simulink model "simulink_model_original"  (R2025a)
settings: Solver=VariableStepAuto  StartTime=0.0  StopTime=10.0  MaxStep=0.2  RelTol=1e-3  AbsTol=1e-3  EnableMultiTasking=on
libraries: fl_lib x8, nesl_utility x6, MyLib_lib x3, simulink x1
CloseFcn:
  | try,close(h1_MechanicalRotationalSystemWithStickSlipMotion),end
  | clear h1_MechanicalRotationalSystemWithStickSlipMotion
  | clear simlog_MechanicalRotationalSystemWithStickSlipMotion
Description:
  | Mechanical Rotational System with Stick-Slip Motion
settings Model: Creator=The MathWorks, Inc.  LastModifiedBy=tbe
settings SolverCC: AutoScaleAbsTol=off  AlgebraicLoopSolver=TrustRegion  MaxZcPerStep=1.0
settings DataIOCC: LimitDataPoints=on  SaveFormat=Array  ReturnWorkspaceOutputs=off
settings OptimizationCC: LifeSpan=inf
settings DebuggingCC: SolverPrmCheckMsg=warning  UnconnectedInputMsg=warning  UnconnectedOutputMsg=warning  UnconnectedLineMsg=warning  AllowSymbolicDim=off  PregeneratedLibrarySubsystemCodeDiagnostic=none  SFUnexpectedBacktrackingDiag=warning  SFNoUnconditionalDefaultTransitionDiag=warning  SFExecutionAtInitializationDiag=none  ArithmeticOperatorsInVariantConditions=warning
settings HardwareCC: ProdBitPerPointer=32.0  ProdBitPerSizeT=32.0  ProdBitPerPtrDiffT=32.0  ProdLargestAtomicFloat=None  ProdIntDivRoundTo=Undefined  ProdEndianess=Unspecified  ProdWordSize=32.0  ProdHWDeviceType=32-bit Generic
settings ModelReferenceCC: EnableRefExpFcnMdlSchedulingChecks=on  PropagateSignalLabelsOutOfModel=off
settings SFSimCC: SimUseLocalCustomCode=off  CustomCodeUndefinedFunction=UseInterfaceOnly
settings RTWCC: RTWUseLocalCustomCode=off  GPUComputeCapability=3.5  DLArmComputeVersion=19.05
settings CodeAppCC: StateflowObjectComments=on
settings GRTTargetCC: TargetLangStandard=C89/C90 (ANSI)
settings ConfigComp: CovMetricSettings=dw  CovSaveCumulativeToWorkspaceVar=on  CovSaveSingleToWorkspaceVar=on  CovExternalEMLEnable=off  CovSFcnEnable=off
settings SimscapeCC: SimscapeLogType=all  SimscapeLogSimulationStatistics=on  SimscapeLogName=simlog_MechanicalRotationalSystemWithStickSlipMotion  SimscapeLogDataHistory=10000.0

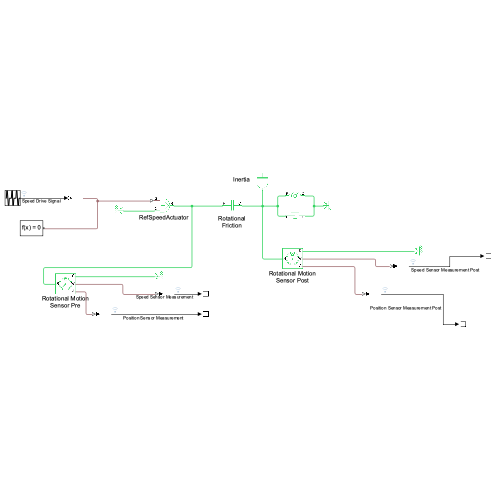
[thumbnail: Simulink's stored preview of the top-level diagram]
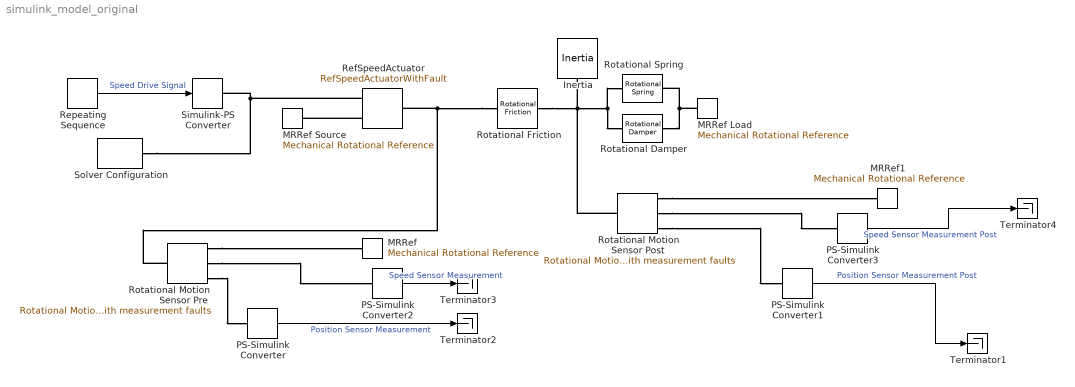
== system simulink_model_original ==
  Inertia : fl_lib/Mechanical/Rotational Elements/Inertia  Tag=Factory Generic  inertia=0.0001 kg*m^2  num_ports=foundation.enum.numPorts2.one  w_specify=off  w_priority=High  w=0 rad/s  w_nominal_specify=off  w_nominal_value=1  w_nominal_unit=rad/s  t_specify=off  t_priority=High  t=0 N*m  t_nominal_specify=off  t_nominal_value=1  t_nominal_unit=N*m
  MRRef : fl_lib/Mechanical/Rotational Elements/Mechanical Rotational Reference  Tag=Factory Generic
  MRRef Load : fl_lib/Mechanical/Rotational Elements/Mechanical Rotational Reference  Tag=Factory Generic
  MRRef Source : fl_lib/Mechanical/Rotational Elements/Mechanical Rotational Reference  Tag=Factory Generic
  MRRef1 : fl_lib/Mechanical/Rotational Elements/Mechanical Rotational Reference  Tag=Factory Generic
  PS-Simulink Converter{,1..3} (4 alike) : nesl_utility/PS-Simulink Converter  PhysicalDomain=network_engine_domain  SubClassName=ps_output  LeftPortType=input  RightPortType=output  PseudoPeriodic=off  Frequencies=[]  VectorFormat=1-D array  Unit=1  AffineConversion=off
  RefSpeedActuator : MyLib_lib/RefSpeedActuatorWithFault  fault_speed_bias=0 rad/s  fault_drift_rate=0 rad/s^2
      settings: InternalSimscapePortConfiguration="{\"Bottom\":[],\"Left\":[{\"id\":\"R\",\"label\":\"R\",\"type\":\"foundation.mechanical.rotational.rotational\"}],\"Right\":[{\"id\":\"S\",\"label\":\"S\",\"type\":\"input\"},{\"id\":\"C\",\"label\":\"C\",\"type\":\"foundation.mechanical.rotational.rotational\"}],\"Top\":[]}"
  Repeating Sequence : simulink/Sources/Repeating Sequence  rep_seq_t=[0 0.98 2 3 4.98 6 7 10]  rep_seq_y=[0 0 6 6 -6 -6 0 0]
  Rotational Friction : fl_lib/Mechanical/Rotational Elements/Rotational Friction  Tag=Factory Generic  brkwy_trq=25 m*N  brkwy_vel=0.06035 rad/s  Col_trq=20 m*N  visc_coef=0.001 m*s*N/rad  w_specify=off  w_priority=High  w=0 rad/s  w_nominal_specify=off  w_nominal_value=1  w_nominal_unit=rad/s  t_specify=off  t_priority=High  t=0 N*m  t_nominal_specify=off  t_nominal_value=1  t_nominal_unit=N*m
  Rotational Damper : fl_lib/Mechanical/Rotational Elements/Rotational Damper  Tag=Factory Generic  D=0.01 m*s*N/rad  w_specify=off  w_priority=High  w=0 rad/s  w_nominal_specify=off  w_nominal_value=1  w_nominal_unit=rad/s  t_specify=off  t_priority=High  t=0 N*m  t_nominal_specify=off  t_nominal_value=1  t_nominal_unit=N*m
  Rotational Motion Sensor Post : MyLib_lib/Rotational Motion Sensor with measurement faults  fault_speed_bias=0 rad/s  fault_speed_gain=0  fault_drift_rate=0 rad/s^2  fault_accel_bias=0 rad/s^2  reference=foundation.enum.MeasurementReference.difference  acceleration_port=false  velocity_port=true  position_port=true  wrap_angle=false  offset=0 rad
      settings: InternalSimscapePortConfiguration="{\"Bottom\":[],\"Left\":[{\"id\":\"R\",\"label\":\"R\",\"type\":\"foundation.mechanical.rotational.rotational\"}],\"Right\":[{\"id\":\"C\",\"label\":\"C\",\"type\":\"foundation.mechanical.rotational.rotational\"},{\"id\":\"W\",\"label\":\"W\",\"type\":\"output\"},{\"id\":\"A\",\"label\":\"A\",\"type\":\"output\"}],\"Top\":[]}"
  Rotational Motion Sensor Pre : MyLib_lib/Rotational Motion Sensor with measurement faults  fault_speed_bias=0 rad/s  fault_speed_gain=0  fault_drift_rate=0 rad/s^2  fault_accel_bias=0 rad/s^2  reference=foundation.enum.MeasurementReference.difference  acceleration_port=false  velocity_port=true  position_port=true  wrap_angle=false  offset=0 rad
      settings: InternalSimscapePortConfiguration="{\"Bottom\":[],\"Left\":[{\"id\":\"R\",\"label\":\"R\",\"type\":\"foundation.mechanical.rotational.rotational\"}],\"Right\":[{\"id\":\"C\",\"label\":\"C\",\"type\":\"foundation.mechanical.rotational.rotational\"},{\"id\":\"W\",\"label\":\"W\",\"type\":\"output\"},{\"id\":\"A\",\"label\":\"A\",\"type\":\"output\"}],\"Top\":[]}"
  Rotational Spring : fl_lib/Mechanical/Rotational Elements/Rotational Spring  Tag=Factory Generic  spr_rate=6.5 N*m/rad  w_specify=off  w_priority=High  w=0 rad/s  w_nominal_specify=off  w_nominal_value=1  w_nominal_unit=rad/s  t_specify=off  t_priority=High  t=0 N*m  t_nominal_specify=off  t_nominal_value=1  t_nominal_unit=N*m  phi_specify=off  phi_priority=High  phi=0 rad  phi_nominal_specify=off  phi_nominal_value=1  phi_nominal_unit=rad
  Simulink-PS Converter : nesl_utility/Simulink-PS Converter  PhysicalDomain=network_engine_domain  SubClassName=ps_input  LeftPortType=input  RightPortType=output  PseudoPeriodic=off  Frequencies=[]  NoiseDistribution=none  NoiseParameters=[]  Unit=1  AffineConversion=off  FilteringAndDerivatives=zero  SimscapeFilterOrder=1  InputFilterTimeConstant=.001  UdotUserProvided=[]
  Solver Configuration : nesl_utility/Solver Configuration  PhysicalDomain=network_engine_domain  SubClassName=solver  LeftPortType=input  RightPortType=generic  Tones=[]  Harmonics=[]  SimulateNoise=off  Profile=off  UseLocalSampling=off  EnableSwitchedLinearOptims=on  FrequencyDomain=off  UseCCode=off  RelTol=0.001  AbsTol=1e-06  MinStep=1e-09  ToWorkspace=off  RevertToSquareIcSolve=off  NumHomotopyIterations=100  PhasorMode=off  PhasorModeNumHarmonics=1  ConsistencySolver=NEWTON_XTOL_AFTER_FTOL  IndexReductionMethod=DerivativeReplacement  DoDC=off  ResidualTolerance=1e-9  ConsistencyTolSource=GLOBAL  ConsistencyAbsTol=0.001  ConsistencyRelTol=0.001  ConsistencyTolFactor=0.001  UseLocalSolver=off  LocalSolverChoice=NE_BACKWARD_EULER_ADVANCER  ResolveIndetEquations=on  FunctionEvalNumThread=1  LocalSolverSampleTime=.001  DoFixedCost=off  MaxNonlinIter=3  MaxModeIter=2  ComputeImpulses=off  ImpulseIterations=2  LinearAlgebra=auto  LinearAlgebraNumThread=0  EquationFormulation=NE_TIME_EF  DelaysMemoryBudget=1024  AutomaticFiltering=on  FilteringTimeConstant=0.001  PartitionStorageMethod=AS_NEEDED  PartitionMemoryBudget=1024  PartitionMethod=FAST  MultibodyUseLocalSolver=off  MultibodyLocalSolverChoice=ODE1  MultibodyLocalSolverSampleTime=0.001
  Terminator{1..4} (4 alike) : Terminator
  wires:
  PS-Simulink Converter/1 -> Terminator2/1  "Position Sensor Measurement"
  PS-Simulink Converter1/1 -> Terminator1/1  "Position Sensor Measurement Post"
  Repeating Sequence/1 -> Simulink-PS Converter/1  "Speed Drive Signal"
  PS-Simulink Converter2/1 -> Terminator3/1  "Speed Sensor Measurement"
  PS-Simulink Converter3/1 -> Terminator4/1  "Speed Sensor Measurement Post"
  connections:
  Rotational Spring/RConn1 -- MRRef Load/LConn1 -- Rotational Damper/RConn1
  Inertia/LConn1 -- Rotational Motion Sensor Post/LConn1 -- Rotational Friction/RConn1 -- Rotational Spring/LConn1 -- Rotational Damper/LConn1
  Rotational Friction/LConn1 -- Rotational Motion Sensor Pre/LConn1 -- RefSpeedActuator/LConn1
  RefSpeedActuator/RConn2 -- MRRef Source/LConn1
  Rotational Motion Sensor Pre/RConn1 -- MRRef/LConn1
  Rotational Motion Sensor Pre/RConn3 -- PS-Simulink Converter/LConn1
  Rotational Motion Sensor Post/RConn3 -- PS-Simulink Converter1/LConn1
  Rotational Motion Sensor Post/RConn1 -- MRRef1/LConn1
  Rotational Motion Sensor Post/RConn2 -- PS-Simulink Converter3/LConn1
  Solver Configuration/RConn1 -- RefSpeedActuator/RConn1 -- Simulink-PS Converter/RConn1
  Rotational Motion Sensor Pre/RConn2 -- PS-Simulink Converter2/LConn1
